simulink model "five_pole"  (R2025a)
settings: Solver=VariableStepAuto  StartTime=0.0  StopTime=20  RelTol=1e-3
undefined symbols (not defined in the file): alpha, beta, Ci, Ji, Jp, Ki5, Kp5, leff, wn
settings Model: Creator=julianshah  LastModifiedBy=julianshah

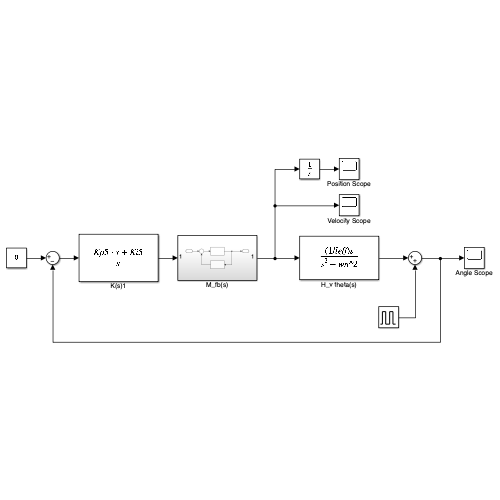
[thumbnail: Simulink's stored preview of the top-level diagram]
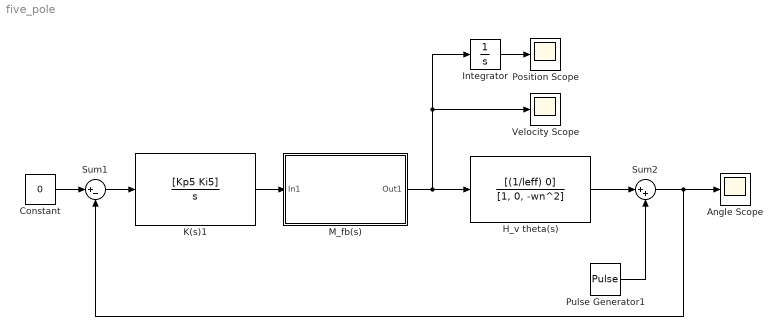
== system five_pole ==
  Angle Scope : Scope
      settings: ActiveDisplayYMinimum=-4.3257846117544858  ActiveDisplayYMaximum=6.92112378186952
  Constant : Constant  Value=0
  H_v theta(s) : TransferFcn  Numerator=[(1/leff) 0]  Denominator=[1, 0, -wn^2]
  Integrator : Integrator
  K(s)1 : TransferFcn  Numerator=[Kp5 Ki5]  Denominator=[1, 0]
  M_fb(s) : Subsystem
  Position Scope : Scope
      settings: ActiveDisplayYMinimum=-2.5148982566220814  ActiveDisplayYMaximum=9.3453502324960418  DataLoggingVariableName=ScopeData2
  Pulse Generator1 : DiscretePulseGenerator  PulseType=Time based  Period=100  PulseWidth=.5
  Sum1 : Sum  Inputs=|+-
  Sum2 : Sum  Inputs=|++
  Velocity Scope : Scope
      settings: ActiveDisplayYMinimum=-13.601525068299406  ActiveDisplayYMaximum=23.708589102320364
  wires:
  Constant/1 -> Sum1/1
  Sum2/1 -> Angle Scope/1, Sum1/2
  Pulse Generator1/1 -> Sum2/2
  Sum1/1 -> K(s)1/1
  K(s)1/1 -> M_fb(s)/1(In1)
  M_fb(s)/1(Out1) -> Velocity Scope/1, Integrator/1, H_v theta(s)/1
  Integrator/1 -> Position Scope/1
  H_v theta(s)/1 -> Sum2/1

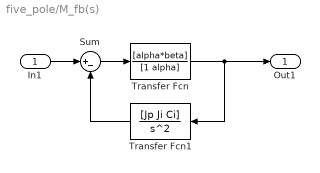
== system five_pole/M_fb(s) ==
  In1 : Inport
  Sum : Sum  Inputs=|+-
  Transfer Fcn : TransferFcn  Numerator=[alpha*beta]  Denominator=[1 alpha]
  Transfer Fcn1 : TransferFcn  Numerator=[Jp Ji Ci]  Denominator=[1 0 0]
  Out1 : Outport
  wires:
  Transfer Fcn/1 -> Transfer Fcn1/1, Out1/1
  Sum/1 -> Transfer Fcn/1
  In1/1 -> Sum/1
  Transfer Fcn1/1 -> Sum/2
